simulink model "mass_spring_damper"  (R2023b)
settings: Solver=VariableStepAuto  StartTime=0.0  StopTime=10.0  RelTol=1e-3
settings Model: Creator=emirh  LastModifiedBy=emirh

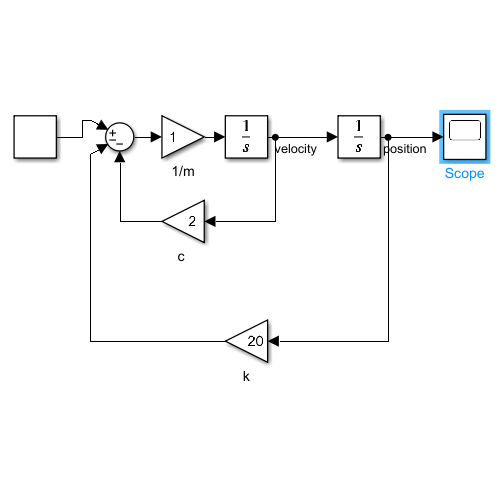
[thumbnail: Simulink's stored preview of the top-level diagram]
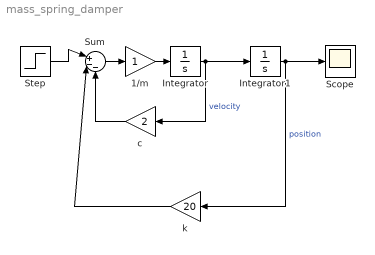
== system mass_spring_damper ==
  1/m : Gain
  Integrator : Integrator
  Integrator1 : Integrator
  Scope : Scope
  Step : Step  Time=0  SampleTime=0
  Sum : Sum  Inputs=|+--
  "c " : Gain  Gain=2
  k : Gain  Gain=20
  wires:
  Step/1 -> Sum/1
  Sum/1 -> 1/m/1
  1/m/1 -> Integrator/1
  Integrator/1 -> "c "/1, Integrator1/1  "velocity"
  Integrator1/1 -> k/1, Scope/1  "position"
  k/1 -> Sum/2
  "c "/1 -> Sum/3
